simulink subsystem "Day1_Scenario_1"  (R2024a)
settings: Solver=VariableStepAuto  StartTime=0.0  StopTime=10.0  RelTol=1e-3
libraries: CarMaker4SL x1
settings Model: Creator=junhyung.cha  LastModifiedBy=pc

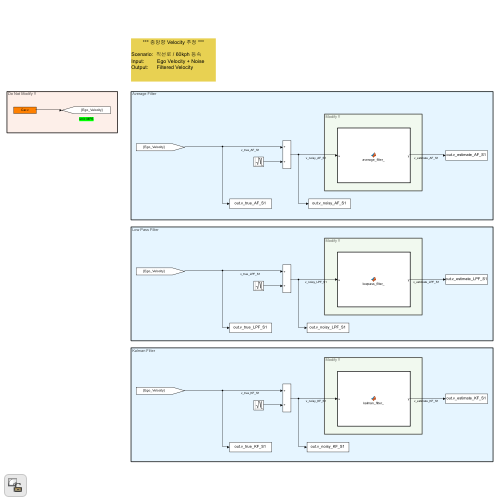
[thumbnail: Simulink's stored preview of the top-level diagram]
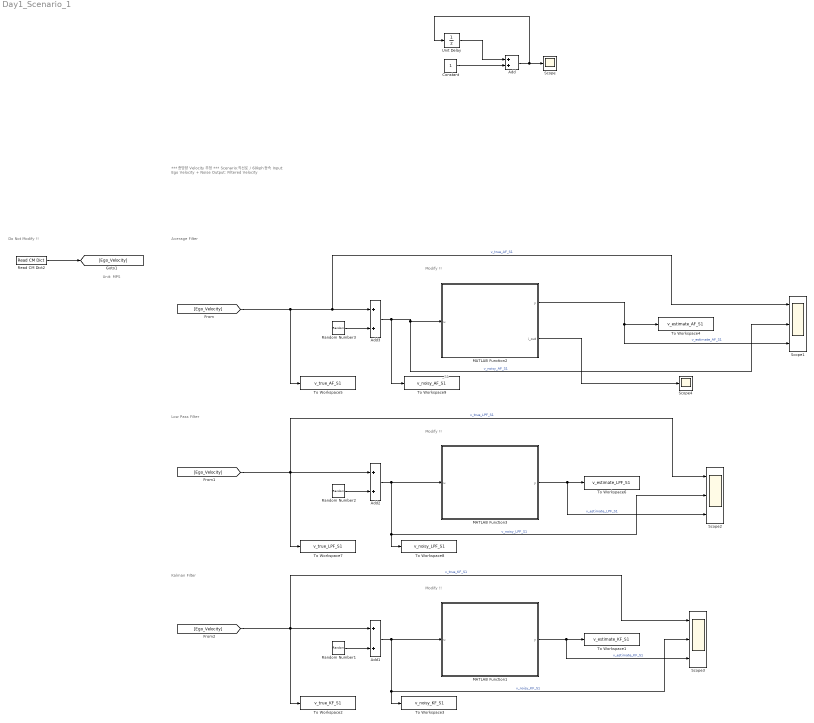
== system Day1_Scenario_1 ==
  note: _S1
  note: Modify !!
  note: Modify !!
  note: Modify !!
  note: Average Filter
  note: Low Pass Filter
  note: Kalman Filter
  note: *** 종방향 Velocity 추정 ***
      |
      | Scenario: 직선로 / 60kph 등속
      | Input: Ego Velocity + Noise
      | Output: Filtered Velocity
  note: Do Not Modify !!
  note: Unit: MPS
  Add{,1..3} (4 alike) : Sum
  Constant : Constant  SampleTime=-1
  MATLAB Function1 : MATLAB Function  TreatAsAtomicUnit=on
  MATLAB Function2 : MATLAB Function  TreatAsAtomicUnit=on
  MATLAB Function3 : MATLAB Function  TreatAsAtomicUnit=on
  Random Number1 : RandomNumber
  Random Number2 : RandomNumber
  Random Number3 : RandomNumber
  Read CM Dict2 : CarMaker4SL/Read CM Dict  xname=Car.v  xsync=off  xstime=Inherited
  Scope : Scope
  Scope1 : Scope  NumInputPorts=3
  Scope2 : Scope  NumInputPorts=3
  Scope3 : Scope  NumInputPorts=3
  Scope4 : Scope
  To Workspace1 : ToWorkspace  VariableName=v_estimate_KF_S1  SaveFormat=Timeseries  SampleTime=-1
  To Workspace2 : ToWorkspace  VariableName=v_true_KF_S1  SaveFormat=Timeseries  SampleTime=-1
  To Workspace3 : ToWorkspace  VariableName=v_noisy_KF_S1  SaveFormat=Timeseries  SampleTime=-1
  To Workspace4 : ToWorkspace  VariableName=v_estimate_AF_S1  SaveFormat=Timeseries  SampleTime=-1
  To Workspace5 : ToWorkspace  VariableName=v_true_AF_S1  SaveFormat=Timeseries  SampleTime=-1
  To Workspace6 : ToWorkspace  VariableName=v_estimate_LPF_S1  SaveFormat=Timeseries  SampleTime=-1
  To Workspace7 : ToWorkspace  VariableName=v_true_LPF_S1  SaveFormat=Timeseries  SampleTime=-1
  To Workspace8 : ToWorkspace  VariableName=v_noisy_LPF_S1  SaveFormat=Timeseries  SampleTime=-1
  To Workspace9 : ToWorkspace  VariableName=v_noisy_AF_S1  SaveFormat=Timeseries  SampleTime=-1
  Unit Delay : UnitDelay  SampleTime=-1  HasFrameUpgradeWarning=on
  wires:
  Random Number2/1 -> Add2/2
  [Ego_Velocity] -> Add2/1, Scope2/1, To Workspace7/1  "v_true_LPF_S1"
  Add2/1 -> MATLAB Function3/1(u), Scope2/2, To Workspace8/1  "v_noisy_LPF_S1"
  MATLAB Function3/1(y) -> To Workspace6/1, Scope2/3  "v_estimate_LPF_S1"
  [Ego_Velocity] -> Add1/1, Scope3/1, To Workspace2/1  "v_true_KF_S1"
  MATLAB Function1/1(y) -> To Workspace1/1, Scope3/3  "v_estimate_KF_S1"
  Random Number1/1 -> Add1/2
  Add1/1 -> MATLAB Function1/1(u), To Workspace3/1, Scope3/2  "v_noisy_KF_S1"
  MATLAB Function2/1(y) -> To Workspace4/1, Scope1/3  "v_estimate_AF_S1"
  Random Number3/1 -> Add3/2
  [Ego_Velocity] -> Add3/1, Scope1/1, To Workspace5/1  "v_true_AF_S1"
  Add3/1 -> MATLAB Function2/1(u), Scope1/2, To Workspace9/1  "v_noisy_AF_S1"
  Read CM Dict2/1 -> [Ego_Velocity]
  Constant/1 -> Add/2
  Unit Delay/1 -> Add/1
  Add/1 -> Scope/1, Unit Delay/1
  MATLAB Function2/2(i_out) -> Scope4/1

== matlab function Day1_Scenario_1/MATLAB Function2 ==
  settings: updateMethod=DISCRETE  sampleTime=0.05
  data: u input; y output; i_out output
function [y,i_out] = average_filter_(u)
%#codegen

    % 윈도우 크기 정의
    N = 20;


    % persistent 변수 선언 (상태 저장용)
    persistent buffer index count i 


    if isempty(buffer)
        buffer = zeros(1, N);
        index = 1;
        count = 0;

    end

    if isempty(i)
        i = 0;
    end

    i = i +1;
    i_out = i;

    if i > 10
        i = 0;
    end

    % 새로운 입력 저장
    buffer(index) = u;
    index = index + 1;

    % 인덱스 순환
    if index > N
        index = 1;
    end

    % 유효한 샘플 수 갱신
    if count < N
        count = count + 1;
    end

    % 평균 계산
    y = sum(buffer) / count;
    
end

== matlab function Day1_Scenario_1/MATLAB Function3 ==
  settings: updateMethod=DISCRETE  sampleTime=0.05
  data: u input; y output
function y = average_filter_(u)
%#codegen

    % 필터 계수
    alpha = 0.1;

    % 이전 출력값 저장용
    persistent y_prev

    % 초기화
    if isempty(y_prev)
        y_prev = u;
    end

    % 1차 저역통과 필터 적용
    y = alpha * u + (1 - alpha) * y_prev;

    % 현재 출력값을 다음 반복을 위한 이전값으로 저장
    y_prev = y;
end

== matlab function Day1_Scenario_1/MATLAB Function1 ==
  settings: updateMethod=DISCRETE  sampleTime=0.05
  data: u input; y output
function y = basic_kalman_filter_(u)
%#codegen
% BASIC_KALMAN_FILTER_  1-D discrete-time Kalman filter
%
%   y = basic_kalman_filter_(u)
%
%   입력:
%     u – 센서로부터 들어오는 측정값
%   출력:
%     y – 칼만 필터로 추정한 상태(estimate_KF)
%
%   내부 모델:
%       x[k] = F*x[k-1]             + w[k-1],   w~N(0,Q)
%       u[k] = H*x[k]               + v[k],     v~N(0,R)
%       y = x  (1-D 상태를 그대로 출력)
%
%   여기서 F = I + A*dt, H = C 로 이산화한 뒤,
%   상태 x 를 직접 출력하는 형태입니다.

    %% 1) 고정 파라미터 정의
    dt = 0.1;       % 샘플링 시간
    A  = 0;         % 연속시간 시스템 계수 A (여기서는 1-D, xdot = A x → A=0 이면 x 불변)
    C  = 1;         % 관측 매트릭스(1×1)
    Q  = 0.01;      % 프로세스 잡음 공분산
    R  = 10;        % 측정 잡음 공분산

    %% 2) persistent 변수 (상태 및 공분산) 초기화
    persistent x_prev P F H
    if isempty(x_prev)
        x_prev = 0;              % 초기 상태 추정치
        P      = 1;              % 초기 오차 공분산
        F      = 1 + A*dt;       % 이산화된 상태 전이 계수
        H      = C;              % 관측 계수
    end

    %% 3) 예측 단계 (Time Update)
    x_pred = F * x_prev;
    P_pred = F * P * F' + Q;

    %% 4) 측정 업데이트 단계 (Measurement Update)
    K      = P_pred * H' / (H * P_pred * H' + R);    % 칼만 이득 계산
    x_upd  = x_pred + K * (u - H * x_pred);           % 상태 추정 갱신
    P      = (1 - K * H) * P_pred;                    % 공분산 갱신

    %% 5) 결과 저장 및 출력
    x_prev = x_upd;
    y      = x_upd;    % 1-D 상태를 그대로 출력
end
